simulink model "sl_robot_sincrono_control_pto"  (R2016b)
settings: Solver=VariableStepAuto  StartTime=0.0  StopTime=tsim  RelTol=1e-3
values from neighbouring files (symbols this model uses):
  omega_sat = [-0.2618 0.2618]    [pruebas_control_P2.m]
  pos_init = [0;0;0]    [pruebas_control_P2.m]
  tetha_d_sat = [-0.75 0.75]    [pruebas_control_P2.m]
  x_ref = in(1)    [control_persecucion.m]    (also in control_pto.m; generador_tray.m = t/100; pruebas_control_P2.m = input(selection))
  y_ref = in(2)    [control_persecucion.m]    (also in control_pto.m; generador_tray.m = 0.1*sin(2*pi*x_ref); pruebas_control_P2.m = input(selection))
settings Model: Creator=marrcogrova  LastModifiedBy=marrcogrova

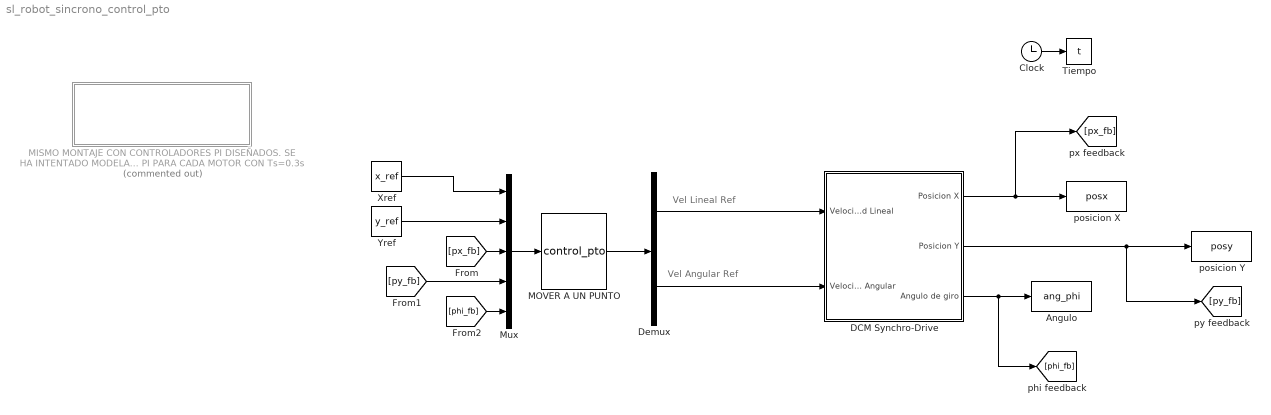
== system sl_robot_sincrono_control_pto ==
  note: Vel Lineal Ref
  note: Vel Angular Ref
  Angulo : ToWorkspace  VariableName=ang_phi  SampleTime=-1
  Clock : Clock
  DCM Synchro-Drive : Subsystem
  Demux : Demux  Outputs=2
  MISMO MONTAJE CON CONTROLADORES PI DISEÑADOS. SE HA INTENTADO MODELAR LOS MOTORES Y DISEÑAR UN PI PARA CADA MOTOR CON Ts=0.3s : Subsystem  Commented=on
  MOVER A UN PUNTO : MATLABFcn  MATLABFcn=control_pto  OutputDimensions=2
  Mux : Mux  Inputs=5
  Tiempo : ToWorkspace  VariableName=t  SampleTime=-1
  Xref : Constant  Value=x_ref
  Yref : Constant  Value=y_ref
  posicion X : ToWorkspace  VariableName=posx  SampleTime=-1
  posicion Y : ToWorkspace  VariableName=posy  SampleTime=-1
  wires:
  Clock/1 -> Tiempo/1
  DCM Synchro-Drive/2(Posicion Y) -> [py_fb], posicion Y/1
  MOVER A UN PUNTO/1 -> Demux/1
  Mux/1 -> MOVER A UN PUNTO/1
  Xref/1 -> Mux/1
  Yref/1 -> Mux/2
  DCM Synchro-Drive/1(Posicion X) -> [px_fb], posicion X/1
  DCM Synchro-Drive/3(Angulo de giro) -> [phi_fb], Angulo/1
  Demux/1 -> DCM Synchro-Drive/1(Velocidad Lineal)
  Demux/2 -> DCM Synchro-Drive/2(Velocidad Angular)
  [px_fb] -> Mux/3
  [py_fb] -> Mux/4
  [phi_fb] -> Mux/5

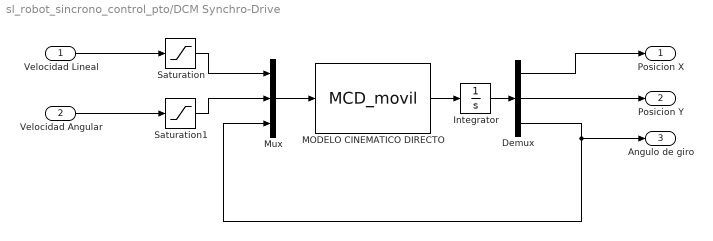
== system sl_robot_sincrono_control_pto/DCM Synchro-Drive ==
  Velocidad Lineal : Inport
  Velocidad Angular : Inport  Port=2
  Demux : Demux  Outputs=3
  Integrator : Integrator  InitialCondition=pos_init
  MODELO CINEMATICO DIRECTO : MATLABFcn  MATLABFcn=MCD_movil  OutputDimensions=3
  Mux : Mux  Inputs=3
  Saturation : Saturate  UpperLimit=tetha_d_sat(2)  LowerLimit=tetha_d_sat(1)
  Saturation1 : Saturate  UpperLimit=omega_sat(2)  LowerLimit=omega_sat(1)
  Posicion X : Outport
  Posicion Y : Outport  Port=2
  Angulo de giro : Outport  Port=3
  wires:
  Integrator/1 -> Demux/1
  Demux/3 -> Angulo de giro/1, Mux/3
  Demux/1 -> Posicion X/1
  Demux/2 -> Posicion Y/1
  Mux/1 -> MODELO CINEMATICO DIRECTO/1
  MODELO CINEMATICO DIRECTO/1 -> Integrator/1
  Velocidad Lineal/1 -> Saturation/1
  Saturation/1 -> Mux/1
  Saturation1/1 -> Mux/2
  Velocidad Angular/1 -> Saturation1/1

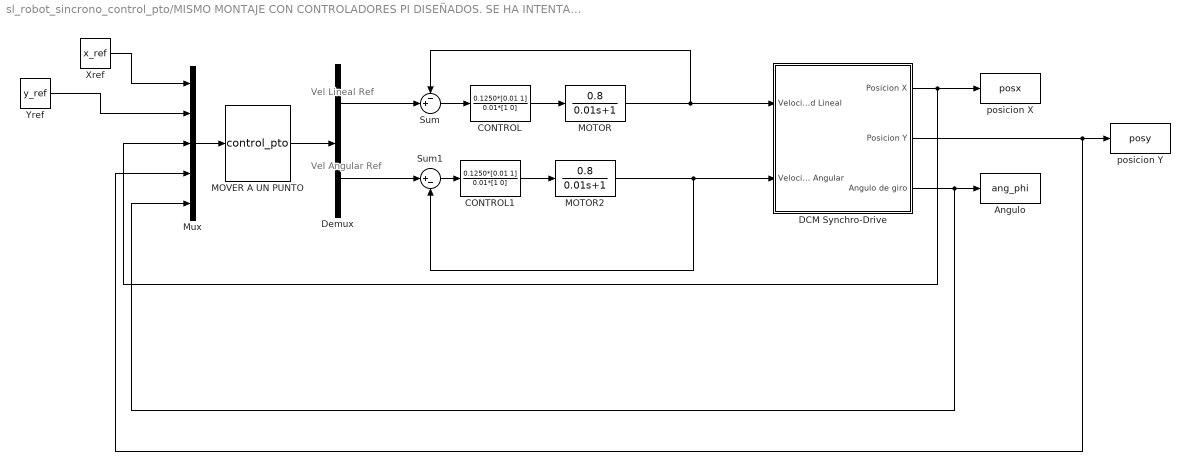
== system sl_robot_sincrono_control_pto/MISMO MONTAJE CON CONTROLADORES PI DISEÑADOS. SE HA INTENTADO MODELAR LOS MOTORES Y DISEÑAR UN PI PARA CADA MOTOR CON Ts=0.3s ==
  note: Vel Lineal Ref
  note: Vel Angular Ref
  Angulo : ToWorkspace  VariableName=ang_phi  SampleTime=-1
  CONTROL : TransferFcn  Numerator=0.1250*[0.01 1]  Denominator=0.01*[1 0]
  CONTROL1 : TransferFcn  Numerator=0.1250*[0.01 1]  Denominator=0.01*[1 0]
  DCM Synchro-Drive : Subsystem
  Demux : Demux  Outputs=2
  MOTOR : TransferFcn  Numerator=0.8  Denominator=[0.01 1]
  MOTOR2 : TransferFcn  Numerator=0.8  Denominator=[0.01 1]
  MOVER A UN PUNTO : MATLABFcn  MATLABFcn=control_pto  OutputDimensions=2
  Mux : Mux  Inputs=5
  Sum : Sum  Inputs=-+|
  Sum1 : Sum  Inputs=|+-
  Xref : Constant  Value=x_ref
  Yref : Constant  Value=y_ref
  posicion X : ToWorkspace  VariableName=posx  SampleTime=-1
  posicion Y : ToWorkspace  VariableName=posy  SampleTime=-1
  wires:
  DCM Synchro-Drive/2(Posicion Y) -> Mux/4, posicion Y/1
  MOVER A UN PUNTO/1 -> Demux/1
  Mux/1 -> MOVER A UN PUNTO/1
  Xref/1 -> Mux/1
  Yref/1 -> Mux/2
  DCM Synchro-Drive/1(Posicion X) -> Mux/3, posicion X/1
  DCM Synchro-Drive/3(Angulo de giro) -> Mux/5, Angulo/1
  Demux/1 -> Sum/2
  Sum/1 -> CONTROL/1
  Demux/2 -> Sum1/1
  Sum1/1 -> CONTROL1/1
  MOTOR2/1 -> DCM Synchro-Drive/2(Velocidad Angular), Sum1/2
  MOTOR/1 -> Sum/1, DCM Synchro-Drive/1(Velocidad Lineal)
  CONTROL/1 -> MOTOR/1
  CONTROL1/1 -> MOTOR2/1

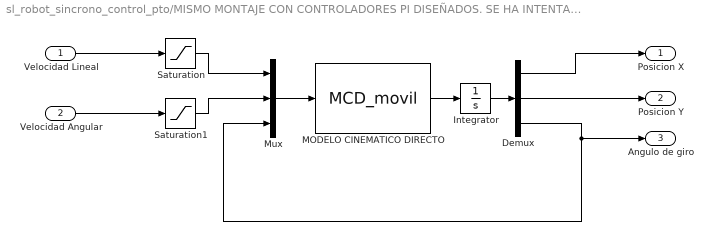
== system sl_robot_sincrono_control_pto/MISMO MONTAJE CON CONTROLADORES PI DISEÑADOS. SE HA INTENTADO MODELAR LOS MOTORES Y DISEÑAR UN PI PARA CADA MOTOR CON Ts=0.3s/DCM Synchro-Drive ==
  Velocidad Lineal : Inport
  Velocidad Angular : Inport  Port=2
  Demux : Demux  Outputs=3
  Integrator : Integrator
  MODELO CINEMATICO DIRECTO : MATLABFcn  MATLABFcn=MCD_movil  OutputDimensions=3
  Mux : Mux  Inputs=3
  Saturation : Saturate  UpperLimit=tetha_d_sat(2)  LowerLimit=tetha_d_sat(1)
  Saturation1 : Saturate  UpperLimit=omega_sat(2)  LowerLimit=omega_sat(1)
  Posicion X : Outport
  Posicion Y : Outport  Port=2
  Angulo de giro : Outport  Port=3
  wires:
  Integrator/1 -> Demux/1
  Demux/3 -> Angulo de giro/1, Mux/3
  Demux/1 -> Posicion X/1
  Demux/2 -> Posicion Y/1
  Mux/1 -> MODELO CINEMATICO DIRECTO/1
  MODELO CINEMATICO DIRECTO/1 -> Integrator/1
  Velocidad Lineal/1 -> Saturation/1
  Saturation/1 -> Mux/1
  Saturation1/1 -> Mux/2
  Velocidad Angular/1 -> Saturation1/1
